simulink model "F_18_fixed"  (R2018a)
settings: Solver=VariableStepAuto  StartTime=0.0  StopTime=75  RelTol=1e-3
values from neighbouring files (symbols this model uses):
  C_h_den = [1 50 400 0]    [F_h_Control.mat]
  C_h_num = [0 1028.99472645 514.497363224 41.1597890579]    [F_h_Control.mat]
  C_inner_den = [1 266.967477525 5165.31702802]    [F_Inner_Control.mat]
  C_inner_num = [0 2795.46957557 1375.1892]    [F_Inner_Control.mat]
undefined symbols (not defined in the file or in its folder): C_out_den, C_out_num, P, PlotVtol
ContinueFcn:
  | FT2frfl
settings Model: Creator=sadam  LastModifiedBy=sadam

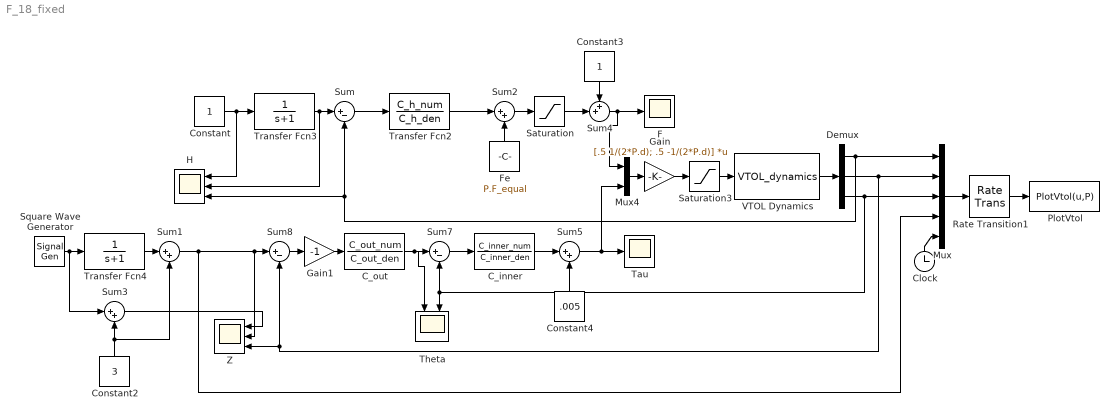
== system F_18_fixed ==
  C_inner : TransferFcn  Numerator=C_inner_num  Denominator=C_inner_den
  C_out : TransferFcn  Numerator=C_out_num  Denominator=C_out_den
  Clock : Clock
  Constant : Constant
  Constant2 : Constant  Value=3
  Constant3 : Constant
  Constant4 : Constant  Value=.005
  Demux : Demux  Outputs=3
  F : Scope
  Fe : Constant  Value=P.F_equal
  Gain : Gain  Gain=[.5 1/(2*P.d); .5 -1/(2*P.d)]  Multiplication=Matrix(K*u)
  Gain1 : Gain  Gain=-1
  "H " : Scope  NumInputPorts=3
  Mux : Mux  Inputs=5
  Mux4 : Mux  Inputs=2
  "PlotVtol " : MATLABFcn  MATLABFcn=PlotVtol(u,P)  OutputDimensions=0
  Rate Transition1 : RateTransition  OutPortSampleTime=P.t_plot
  Saturation : Saturate  UpperLimit=P.Force_max  LowerLimit=-P.Force_max
  Saturation3 : Saturate  UpperLimit=P.Force_max  LowerLimit=-P.Force_max
  Square Wave Generator : SignalGenerator  WaveForm=square  Amplitude=2  Frequency=.05/2
  Sum : Sum  Inputs=|+-
  Sum{1..3,5} (4 alike) : Sum  Inputs=|++
  Sum4 : Sum  Inputs=++|
  Sum7 : Sum  Inputs=|+-
  Sum8 : Sum  Inputs=|+-
  Tau : Scope
  "Theta " : Scope  NumInputPorts=2
  Transfer Fcn2 : TransferFcn  Numerator=C_h_num  Denominator=C_h_den
  Transfer Fcn3 : TransferFcn  Denominator=[1 1]
  Transfer Fcn4 : TransferFcn  Denominator=[1 1]
  VTOL Dynamics : S-Function  FunctionName=VTOL_dynamics  Parameters=P  SFunctionDeploymentMode=off  EnableBusSupport=off
  Z : Scope  NumInputPorts=3
  wires:
  Mux/1 -> Rate Transition1/1
  VTOL Dynamics/1 -> Demux/1
  Rate Transition1/1 -> "PlotVtol "/1
  Sum1/1 -> Z/2, Sum8/1, Mux/4
  Clock/1 -> Mux/5
  Demux/1 -> Mux/1, "H "/3, Sum/2
  Demux/2 -> Mux/2, Z/3, Sum8/2
  Demux/3 -> Mux/3, "Theta "/2, Sum7/2
  Gain/1 -> Saturation3/1
  Mux4/1 -> Gain/1
  Sum2/1 -> Saturation/1
  Fe/1 -> Sum2/2
  Constant2/1 -> Sum1/2, Sum3/2
  Sum/1 -> Transfer Fcn2/1
  Transfer Fcn2/1 -> Sum2/1
  Constant/1 -> "H "/1, Transfer Fcn3/1
  Transfer Fcn3/1 -> "H "/2, Sum/1
  Sum7/1 -> C_inner/1
  C_out/1 -> Sum7/1, "Theta "/1
  Transfer Fcn4/1 -> Sum1/1
  Square Wave Generator/1 -> Sum3/1, Transfer Fcn4/1
  Sum3/1 -> Z/1
  Gain1/1 -> C_out/1
  Sum8/1 -> Gain1/1
  Saturation3/1 -> VTOL Dynamics/1
  Saturation/1 -> Sum4/2
  Sum4/1 -> Mux4/1, F/1
  Constant3/1 -> Sum4/1
  C_inner/1 -> Sum5/1
  Sum5/1 -> Mux4/2, Tau/1
  Constant4/1 -> Sum5/2
